simulink model "test_GRM_Airframe"  (R2019b)
settings: Solver=FixedStepAuto  StartTime=0.0  StopTime=60  FixedStep=0.001  RelTol=1e-3
PreLoadFcn:
  | addpath('init_functions');
  | init_grm;
  | addpath('parameters');
  | para_def_grm;
values from neighbouring files (symbols this model uses):
  a_vBEW = 0    [init_grm.m]
  act_dmp = 0.6322    [para_def_grm.m]
  act_omega = 59.9250    (= 59.925)    [para_def_grm.m]
  aero = load('aero.mat')    [para_def_grm.m]
  c_be = -6.5e-3    (= -0.0065)    [init_grm.m]
  c_h_geop0 = 0    [init_grm.m]
  c_h_geope = 11e3    (= 11000)    [init_grm.m]
  c_pa0 = 101325    [init_grm.m]
  c_pe = -c_g0/c_be/sgc    (= 5.25587981272)    [init_grm.m]
  c_r0 = 6371000.79    [init_grm.m]
  c_rot = 7.292115e-5    (= 7.292115e-05)    [init_grm.m]
  c_Tmp0 = 288.15    [init_grm.m]
  chW = pi/2    (= 1.57079632679)    [init_grm.m]
  D = JD - 2451545.0    [init_grm.m]
  d_siB_0 = 0    [para_def_grm.m]
  d_siB_max = deg2rad(1200)    [para_def_grm.m]
  d_siB_min = deg2rad(-1200)    [para_def_grm.m]
  dd_siB_max = deg2rad(50000)    [para_def_grm.m]
  dd_siB_min = deg2rad(-50000)    [para_def_grm.m]
  de_JBBB_xx = JBBB_xx_0 - JBBB_xx_e    (= 0)    [para_def_grm.m]
  de_JBBB_yy = JBBB_yy_0 - JBBB_yy_e    (= 0)    [para_def_grm.m]
  de_JBBB_zz = JBBB_zz_0 - JBBB_zz_e    (= 0)    [para_def_grm.m]
  de_mM = m_fuel_lookup(end)    [para_def_grm.m]
  e_pa = 0    [init_grm.m]
  e_Tmp = 0    [init_grm.m]
  F_prp = [450.52;428.7;423.25;391.61;352.34;304.35;266.17;243.26;216.92 ... (first row only)    [para_def_grm.m]
  flag_I_aero_switch = 1    [init_grm.m]
  flag_I_flat = 1    [init_grm.m]
  flag_I_gravity_switch = 1    [init_grm.m]
  flag_I_rot = 0    [init_grm.m]
  hcr = 1.4    [init_grm.m]
  J0PB_e = TBP*J0PP_e*TBP'    [para_def_grm.m]
  JMMM_0 = TBP*J0PP_0*TBP'    [para_def_grm.m]
  JMMM_e = TBP*J0PP_e*TBP'    [para_def_grm.m]
  lat_0 = 0    [init_grm.m]
  lon_0 = 0    [init_grm.m]
  m0 = mB_0    (= 3.30977)    [para_def_grm.m]
  m_fuel_lookup = [0;0.0573;0.1127;0.1667;0.2186;0.2681;0.3149;0.3588 ... (first row only)    [para_def_grm.m]
  mB_0 = 3.30977    [para_def_grm.m]
  mM_0 = 1.119    [para_def_grm.m]
  mM_e = de_mM    [para_def_grm.m]
  p0PB = [x0PB;y0PB;z0PB]    [para_def_grm.m]
  pBII_0 = TIE_0*pBEE_0    [init_grm.m]
  pMPB = [xMPB;yMPB;zMPB]    [para_def_grm.m]
  pNPB = [0;0;0]    [para_def_grm.m]
  qEG_0 = q12_from_T12(TEG)    [init_grm.m]
  qIB_0 = qumul(qIG_0,qGB_0)    [init_grm.m]
  qIE_0 = q12_from_T12(TIE_0)    [init_grm.m]
  sgc = 287.05287    [init_grm.m]
  siB_0 = 0    [para_def_grm.m]
  siB_max = deg2rad(30)    [para_def_grm.m]
  siB_min = deg2rad(-30)    [para_def_grm.m]
  t_prp1 = [0.04;0.28;0.54;1;1.48;1.99;2.51;3;3.5;3.67;3.82;4]    [para_def_grm.m]
  t_prp2 = t_prp2'    [para_def_grm.m]
  T_sim_lnch = -5    [init_grm.m]
  Tr3r4 = [1,1,1,1;1,1,-1,-1;-1,1,1,-1]*0.25    [para_def_grm.m]
  Tr4r3 = [1,1,-1;1,1,1;1,-1,1;1,-1,-1]    [para_def_grm.m]
  tRRR = 0    [para_def_grm.m]
  unc_a_vBEW_bl = 0    [para_def_grm.m]
  unc_act_bl = 0    [para_def_grm.m]
  unc_act_off = 0    [para_def_grm.m]
  unc_act_scale = 1    [para_def_grm.m]
  unc_aero_Cl_scale = 1    [para_def_grm.m]
  unc_aero_Cm_scale = 1    [para_def_grm.m]
  unc_aero_Cn_scale = 1    [para_def_grm.m]
  unc_aero_Cx_scale = 1    [para_def_grm.m]
  unc_aero_Cy_scale = 1    [para_def_grm.m]
  unc_aero_Cz_scale = 1    [para_def_grm.m]
  unc_cg_x = 0    [para_def_grm.m]
  unc_cg_y = 0    [para_def_grm.m]
  unc_cg_z = 0    [para_def_grm.m]
  unc_chW_bl = 0    [para_def_grm.m]
  unc_fin_def_pitch = 0    [para_def_grm.m]
  unc_fin_def_roll = 0    [para_def_grm.m]
  unc_fin_def_yaw = 0    [para_def_grm.m]
  unc_mB_bl = 0    [para_def_grm.m]
  unc_mB_scale = 1    [para_def_grm.m]
  unc_moi_Jxx = 0    [para_def_grm.m]
  unc_moi_Jyy = 0    [para_def_grm.m]
  unc_moi_Jzz = 0    [para_def_grm.m]
  unc_prp_scale = 1    [para_def_grm.m]
  unc_prp_x = 0    [para_def_grm.m]
  unc_prp_y = 0    [para_def_grm.m]
  unc_prp_z = 0    [para_def_grm.m]
  vBII_0 = vBEE_0 + cross(wIEI_0,pBII_0)    [init_grm.m]
  wBIB_0 = r2_from_r1_trans_q21(wBII_0,qBI_0)    [init_grm.m]
  x0PB = -0.5    [para_def_grm.m]
  xMPB = -0.9    [para_def_grm.m]
  y0PB = 0    [para_def_grm.m]
  yMPB = 0    [para_def_grm.m]
  z0PB = 0    [para_def_grm.m]
  zMPB = 0    [para_def_grm.m]
undefined symbols (not defined in the file or in its folder): c_b_WGS, c_flat, c_grav, c_rsma, d_mB_lookup, t_dmB
libraries: simulink_extras x14, simulink x3
(part 6 of 6)

== system test_GRM_Airframe/GRM_Airframe/rb_eom/eom_6dof/Rigid_Body_EOM_6_DOF/rb_eom_6dof/r2_from_r1_trans_q21 ==
  note: Outputs [size]:
      |
      | vector r2 [3]
  note: Inputs [size]:
      |
      | vector r1 [3]
      | quaternion q21 [4]
  r1 : Inport
  q21 : Inport  Port=2
  Add : Sum  Inputs=++++
  Add1 : Sum  Inputs=++++
  Constant : Constant  Value=0
  Demux : Demux  Outputs=3
  Demux1 : Demux
  Demux2 : Demux
  Math Function : Math  Operator=transpose  SaturateOnIntegerOverflow=on
  Product{,1..7} (8 alike) : Product
  Product8 : Product  Inputs=3  Multiplication=Matrix(*)
  Q_1 : Constant  Value=[0 0 0 1; 0 0 1 0; 0 -1 0 0; -1 0 0 0]
  Q_2 : Constant  Value=[0 0 -1 0; 0 0 0 1; 1 0 0 0; 0 -1 0 0]
  Q_3 : Constant  Value=[0 1 0 0; -1 0 0 0; 0 0 0 1; 0 0 -1 0]
  Q_4 : Constant  Value=[1 0 0 0; 0 1 0 0; 0 0 1 0; 0 0 0 1]
  Q~_1 : Constant  Value=[0 0 0 1; 0 0 -1 0; 0 1 0 0; -1 0 0 0]
  Q~_2 : Constant  Value=[0 0 1 0; 0 0 0 1; -1 0 0 0; 0 -1 0 0]
  Q~_3 : Constant  Value=[0 -1 0 0; 1 0 0 0; 0 0 0 1; 0 0 -1 0]
  Q~_4 : Constant  Value=[1 0 0 0; 0 1 0 0; 0 0 1 0; 0 0 0 1]
  Selector : Selector  IndexMode=Zero-based  InputPortWidth=4  IndexOptions=Index vector (dialog)  Indices=[0 1 2]  OutputSizes=1
  Vector Concatenate : Concatenate  NumInputs=4
  r2 : Outport  VectorParamsAs1DForOutWhenUnconnected=off
  wires:
  Selector/1 -> r2/1
  Product8/1 -> Selector/1
  Vector Concatenate/1 -> Product8/3
  Constant/1 -> Vector Concatenate/4
  Math Function/1 -> Product8/1  "Q~T(q)"
  Q~_3/1 -> Product6/1
  Q~_1/1 -> Product4/1
  Q~_4/1 -> Product7/1
  Product6/1 -> Add1/3
  Demux2/3 -> Product6/2  "q3"
  Product5/1 -> Add1/2
  Demux2/2 -> Product5/2  "q2"
  Add1/1 -> Math Function/1  "Q~(q)"
  q21/1 -> Demux1/1, Demux2/1
  Product7/1 -> Add1/4
  Product4/1 -> Add1/1
  Q~_2/1 -> Product5/1
  Demux2/4 -> Product7/2  "q4"
  Demux2/1 -> Product4/2  "q1"
  Add/1 -> Product8/2  "Q(q)"
  Product3/1 -> Add/4
  Product2/1 -> Add/3
  Product1/1 -> Add/2
  Product/1 -> Add/1
  Q_4/1 -> Product3/1
  Q_3/1 -> Product2/1
  Q_2/1 -> Product1/1
  Q_1/1 -> Product/1
  Demux1/4 -> Product3/2  "q4"
  Demux1/3 -> Product2/2  "q3"
  Demux1/2 -> Product1/2  "q2"
  Demux1/1 -> Product/2  "q1"
  Demux/3 -> Vector Concatenate/3  "rz"
  Demux/2 -> Vector Concatenate/2  "ry"
  Demux/1 -> Vector Concatenate/1  "rx"
  r1/1 -> Demux/1

== system test_GRM_Airframe/GRM_Airframe/stream_flow/calc_stream_flow/Subsystem1/AoA_Sideslip_Alphatot_Phi/norm_of_vector ==
  note: Outputs [size]:
      |
      | norm of vector [1]
  note: Inputs [size]:
      |
      | vector  [3]
  vector : Inport
  Dot Product1 : DotProduct  InputSameDT=on  OutDataTypeStr=Inherit: Inherit via internal rule
  Math Function1 : Math  Operator=sqrt  SaturateOnIntegerOverflow=on
  norm_of_vector : Outport  VectorParamsAs1DForOutWhenUnconnected=off
  wires:
  vector/1 -> Dot Product1/1, Dot Product1/2
  Math Function1/1 -> norm_of_vector/1
  Dot Product1/1 -> Math Function1/1

== system test_GRM_Airframe/GRM_Airframe/weight_and_balance/moi/moi_coordinate_transformation/3_rot_mat/1. Rotation x-Achse ==
  alpha1 : Inport
  Constant : Constant
  Constant{1..2,7..8} (4 alike) : Constant  Value=0
  Gain : Gain  Gain=-1
  Matrix Concatenate : Concatenate  NumInputs=3  Mode=Multidimensional array  ConcatenateDimension=2
  Mux : Mux  Inputs=3
  Mux1 : Mux  Inputs=3
  Mux2 : Mux  Inputs=3
  Trigonometric Function : Trigonometry  Operator=cos
  Trigonometric Function1 : Trigonometry
  Trigonometric Function2 : Trigonometry
  Trigonometric Function3 : Trigonometry  Operator=cos
  1Rot_Matrix_x : Outport  VectorParamsAs1DForOutWhenUnconnected=off
  wires:
  Gain/1 -> Mux1/3
  alpha1/1 -> Trigonometric Function2/1, Trigonometric Function/1, Trigonometric Function1/1, Trigonometric Function3/1
  Constant/1 -> Mux/1
  Constant1/1 -> Mux/2
  Constant2/1 -> Mux/3
  Constant8/1 -> Mux1/1
  Trigonometric Function/1 -> Mux1/2
  Trigonometric Function2/1 -> Gain/1
  Constant7/1 -> Mux2/1
  Trigonometric Function1/1 -> Mux2/2
  Trigonometric Function3/1 -> Mux2/3
  Mux/1 -> Matrix Concatenate/1
  Mux1/1 -> Matrix Concatenate/2
  Mux2/1 -> Matrix Concatenate/3
  Matrix Concatenate/1 -> 1Rot_Matrix_x/1

== system test_GRM_Airframe/GRM_Airframe/weight_and_balance/moi/moi_coordinate_transformation/3_rot_mat/1. Rotation y-Achse ==
  alpha1 : Inport
  Constant{,2,7..8} (4 alike) : Constant  Value=0
  Constant1 : Constant
  Gain1 : Gain  Gain=-1
  Matrix Concatenate : Concatenate  NumInputs=3  Mode=Multidimensional array  ConcatenateDimension=2
  Mux : Mux  Inputs=3
  Mux1 : Mux  Inputs=3
  Mux2 : Mux  Inputs=3
  Trigonometric Function : Trigonometry  Operator=cos
  Trigonometric Function1 : Trigonometry
  Trigonometric Function2 : Trigonometry
  Trigonometric Function3 : Trigonometry  Operator=cos
  1Rot_Matrix_y : Outport  VectorParamsAs1DForOutWhenUnconnected=off
  wires:
  Gain1/1 -> Mux2/1
  Mux2/1 -> Matrix Concatenate/3
  Mux1/1 -> Matrix Concatenate/2
  Mux/1 -> Matrix Concatenate/1
  Trigonometric Function3/1 -> Mux2/3
  Trigonometric Function1/1 -> Gain1/1
  Constant2/1 -> Mux1/3
  Constant1/1 -> Mux1/2
  Constant/1 -> Mux1/1
  alpha1/1 -> Trigonometric Function1/1, Trigonometric Function3/1, Trigonometric Function2/1, Trigonometric Function/1
  Constant8/1 -> Mux/2
  Trigonometric Function/1 -> Mux/1
  Trigonometric Function2/1 -> Mux/3
  Constant7/1 -> Mux2/2
  Matrix Concatenate/1 -> 1Rot_Matrix_y/1

== system test_GRM_Airframe/GRM_Airframe/weight_and_balance/moi/moi_coordinate_transformation/3_rot_mat/1. Rotation z-Achse ==
  alpha1 : Inport
  Constant{4,7..8,10} (4 alike) : Constant  Value=0
  Constant11 : Constant
  Gain : Gain  Gain=-1
  Matrix Concatenate : Concatenate  NumInputs=3  Mode=Multidimensional array  ConcatenateDimension=2
  Mux : Mux  Inputs=3
  Mux1 : Mux  Inputs=3
  Mux2 : Mux  Inputs=3
  Trigonometric Function : Trigonometry  Operator=cos
  Trigonometric Function1 : Trigonometry
  Trigonometric Function3 : Trigonometry  Operator=cos
  Trigonometric Function4 : Trigonometry
  1Rot_Matrix_z : Outport  VectorParamsAs1DForOutWhenUnconnected=off
  wires:
  Gain/1 -> Mux/2
  Trigonometric Function/1 -> Mux1/2
  Mux/1 -> Matrix Concatenate/1
  Mux1/1 -> Matrix Concatenate/2
  Mux2/1 -> Matrix Concatenate/3
  Trigonometric Function1/1 -> Mux1/1
  Constant7/1 -> Mux1/3
  Constant4/1 -> Mux2/1
  Constant10/1 -> Mux2/2
  Constant11/1 -> Mux2/3
  Trigonometric Function3/1 -> Mux/1
  Trigonometric Function4/1 -> Gain/1
  Constant8/1 -> Mux/3
  Matrix Concatenate/1 -> 1Rot_Matrix_z/1
  alpha1/1 -> Trigonometric Function3/1, Trigonometric Function4/1, Trigonometric Function/1, Trigonometric Function1/1

== system test_GRM_Airframe/GRM_Airframe/weight_and_balance/moi/moi_coordinate_transformation/3_rot_mat/2. Rotation x-Achse ==
  alpha2 : Inport
  Constant : Constant
  Constant{1..2,7..8} (4 alike) : Constant  Value=0
  Gain : Gain  Gain=-1
  Matrix Concatenate : Concatenate  NumInputs=3  Mode=Multidimensional array  ConcatenateDimension=2
  Mux : Mux  Inputs=3
  Mux1 : Mux  Inputs=3
  Mux2 : Mux  Inputs=3
  Trigonometric Function : Trigonometry  Operator=cos
  Trigonometric Function1 : Trigonometry
  Trigonometric Function2 : Trigonometry
  Trigonometric Function3 : Trigonometry  Operator=cos
  2Rot_Matrix_x : Outport  VectorParamsAs1DForOutWhenUnconnected=off
  wires:
  Gain/1 -> Mux1/3
  alpha2/1 -> Trigonometric Function2/1, Trigonometric Function/1, Trigonometric Function1/1, Trigonometric Function3/1
  Constant/1 -> Mux/1
  Constant1/1 -> Mux/2
  Constant2/1 -> Mux/3
  Constant8/1 -> Mux1/1
  Trigonometric Function/1 -> Mux1/2
  Trigonometric Function2/1 -> Gain/1
  Constant7/1 -> Mux2/1
  Trigonometric Function1/1 -> Mux2/2
  Trigonometric Function3/1 -> Mux2/3
  Mux/1 -> Matrix Concatenate/1
  Mux1/1 -> Matrix Concatenate/2
  Mux2/1 -> Matrix Concatenate/3
  Matrix Concatenate/1 -> 2Rot_Matrix_x/1

== system test_GRM_Airframe/GRM_Airframe/weight_and_balance/moi/moi_coordinate_transformation/3_rot_mat/2. Rotation y-Achse ==
  alpha2 : Inport
  Constant{,2,7..8} (4 alike) : Constant  Value=0
  Constant1 : Constant
  Gain1 : Gain  Gain=-1
  Matrix Concatenate : Concatenate  NumInputs=3  Mode=Multidimensional array  ConcatenateDimension=2
  Mux : Mux  Inputs=3
  Mux1 : Mux  Inputs=3
  Mux2 : Mux  Inputs=3
  Trigonometric Function : Trigonometry  Operator=cos
  Trigonometric Function1 : Trigonometry
  Trigonometric Function2 : Trigonometry
  Trigonometric Function3 : Trigonometry  Operator=cos
  2Rot_Matrix_y : Outport  VectorParamsAs1DForOutWhenUnconnected=off
  wires:
  Gain1/1 -> Mux2/1
  Mux2/1 -> Matrix Concatenate/3
  Mux1/1 -> Matrix Concatenate/2
  Mux/1 -> Matrix Concatenate/1
  Trigonometric Function3/1 -> Mux2/3
  Trigonometric Function1/1 -> Gain1/1
  Constant2/1 -> Mux1/3
  Constant1/1 -> Mux1/2
  Constant/1 -> Mux1/1
  alpha2/1 -> Trigonometric Function1/1, Trigonometric Function3/1, Trigonometric Function2/1, Trigonometric Function/1
  Constant8/1 -> Mux/2
  Trigonometric Function/1 -> Mux/1
  Trigonometric Function2/1 -> Mux/3
  Constant7/1 -> Mux2/2
  Matrix Concatenate/1 -> 2Rot_Matrix_y/1

== system test_GRM_Airframe/GRM_Airframe/weight_and_balance/moi/moi_coordinate_transformation/3_rot_mat/2. Rotation z-Achse ==
  alpha2 : Inport
  Constant{4,7..8,10} (4 alike) : Constant  Value=0
  Constant11 : Constant
  Gain : Gain  Gain=-1
  Matrix Concatenate : Concatenate  NumInputs=3  Mode=Multidimensional array  ConcatenateDimension=2
  Mux : Mux  Inputs=3
  Mux1 : Mux  Inputs=3
  Mux2 : Mux  Inputs=3
  Trigonometric Function : Trigonometry  Operator=cos
  Trigonometric Function1 : Trigonometry
  Trigonometric Function3 : Trigonometry  Operator=cos
  Trigonometric Function4 : Trigonometry
  2Rot_Matrix_z : Outport  VectorParamsAs1DForOutWhenUnconnected=off
  wires:
  Gain/1 -> Mux/2
  Trigonometric Function/1 -> Mux1/2
  Mux/1 -> Matrix Concatenate/1
  Mux1/1 -> Matrix Concatenate/2
  Mux2/1 -> Matrix Concatenate/3
  Trigonometric Function1/1 -> Mux1/1
  Constant7/1 -> Mux1/3
  Constant4/1 -> Mux2/1
  Constant10/1 -> Mux2/2
  Constant11/1 -> Mux2/3
  Trigonometric Function3/1 -> Mux/1
  Trigonometric Function4/1 -> Gain/1
  Constant8/1 -> Mux/3
  Matrix Concatenate/1 -> 2Rot_Matrix_z/1
  alpha2/1 -> Trigonometric Function3/1, Trigonometric Function4/1, Trigonometric Function/1, Trigonometric Function1/1

== system test_GRM_Airframe/GRM_Airframe/weight_and_balance/moi/moi_coordinate_transformation/3_rot_mat/3. Rotation x-Achse ==
  alpha3 : Inport
  Constant : Constant
  Constant{1..2,7..8} (4 alike) : Constant  Value=0
  Gain : Gain  Gain=-1
  Matrix Concatenate : Concatenate  NumInputs=3  Mode=Multidimensional array  ConcatenateDimension=2
  Mux : Mux  Inputs=3
  Mux1 : Mux  Inputs=3
  Mux2 : Mux  Inputs=3
  Trigonometric Function : Trigonometry  Operator=cos
  Trigonometric Function1 : Trigonometry
  Trigonometric Function2 : Trigonometry
  Trigonometric Function3 : Trigonometry  Operator=cos
  3Rot_Matrix_x : Outport  VectorParamsAs1DForOutWhenUnconnected=off
  wires:
  Gain/1 -> Mux1/3
  alpha3/1 -> Trigonometric Function2/1, Trigonometric Function/1, Trigonometric Function1/1, Trigonometric Function3/1
  Constant/1 -> Mux/1
  Constant1/1 -> Mux/2
  Constant2/1 -> Mux/3
  Constant8/1 -> Mux1/1
  Trigonometric Function/1 -> Mux1/2
  Trigonometric Function2/1 -> Gain/1
  Constant7/1 -> Mux2/1
  Trigonometric Function1/1 -> Mux2/2
  Trigonometric Function3/1 -> Mux2/3
  Mux/1 -> Matrix Concatenate/1
  Mux1/1 -> Matrix Concatenate/2
  Mux2/1 -> Matrix Concatenate/3
  Matrix Concatenate/1 -> 3Rot_Matrix_x/1

== system test_GRM_Airframe/GRM_Airframe/weight_and_balance/moi/moi_coordinate_transformation/3_rot_mat/3. Rotation y-Achse ==
  alpha3 : Inport
  Constant{,2,7..8} (4 alike) : Constant  Value=0
  Constant1 : Constant
  Gain1 : Gain  Gain=-1
  Matrix Concatenate : Concatenate  NumInputs=3  Mode=Multidimensional array  ConcatenateDimension=2
  Mux : Mux  Inputs=3
  Mux1 : Mux  Inputs=3
  Mux2 : Mux  Inputs=3
  Trigonometric Function : Trigonometry  Operator=cos
  Trigonometric Function1 : Trigonometry
  Trigonometric Function2 : Trigonometry
  Trigonometric Function3 : Trigonometry  Operator=cos
  3Rot_Matrix_y : Outport  VectorParamsAs1DForOutWhenUnconnected=off
  wires:
  Gain1/1 -> Mux2/1
  Mux2/1 -> Matrix Concatenate/3
  Mux1/1 -> Matrix Concatenate/2
  Mux/1 -> Matrix Concatenate/1
  Trigonometric Function3/1 -> Mux2/3
  Trigonometric Function1/1 -> Gain1/1
  Constant2/1 -> Mux1/3
  Constant1/1 -> Mux1/2
  Constant/1 -> Mux1/1
  alpha3/1 -> Trigonometric Function1/1, Trigonometric Function3/1, Trigonometric Function2/1, Trigonometric Function/1
  Constant8/1 -> Mux/2
  Trigonometric Function/1 -> Mux/1
  Trigonometric Function2/1 -> Mux/3
  Constant7/1 -> Mux2/2
  Matrix Concatenate/1 -> 3Rot_Matrix_y/1

== system test_GRM_Airframe/GRM_Airframe/weight_and_balance/moi/moi_coordinate_transformation/3_rot_mat/3. Rotation z-Achse ==
  alpha3 : Inport
  Constant{4,7..8,10} (4 alike) : Constant  Value=0
  Constant11 : Constant
  Gain : Gain  Gain=-1
  Matrix Concatenate : Concatenate  NumInputs=3  Mode=Multidimensional array  ConcatenateDimension=2
  Mux : Mux  Inputs=3
  Mux1 : Mux  Inputs=3
  Mux2 : Mux  Inputs=3
  Trigonometric Function : Trigonometry  Operator=cos
  Trigonometric Function1 : Trigonometry
  Trigonometric Function3 : Trigonometry  Operator=cos
  Trigonometric Function4 : Trigonometry
  3Rot_Matrix_z : Outport  VectorParamsAs1DForOutWhenUnconnected=off
  wires:
  Gain/1 -> Mux/2
  Trigonometric Function/1 -> Mux1/2
  Mux/1 -> Matrix Concatenate/1
  Mux1/1 -> Matrix Concatenate/2
  Mux2/1 -> Matrix Concatenate/3
  Trigonometric Function1/1 -> Mux1/1
  Constant7/1 -> Mux1/3
  Constant4/1 -> Mux2/1
  Constant10/1 -> Mux2/2
  Constant11/1 -> Mux2/3
  Trigonometric Function3/1 -> Mux/1
  Trigonometric Function4/1 -> Gain/1
  Constant8/1 -> Mux/3
  Matrix Concatenate/1 -> 3Rot_Matrix_z/1
  alpha3/1 -> Trigonometric Function3/1, Trigonometric Function4/1, Trigonometric Function/1, Trigonometric Function1/1

== system test_GRM_Airframe/environment_global/weather/atm_dynamic/trafo_around_z_axis/1_rot_mat/1. Rotation x-Achse ==
  alpha1 : Inport
  Constant : Constant
  Constant{1..2,7..8} (4 alike) : Constant  Value=0
  Gain : Gain  Gain=-1
  Matrix Concatenate : Concatenate  NumInputs=3  Mode=Multidimensional array  ConcatenateDimension=2
  Mux : Mux  Inputs=3
  Mux1 : Mux  Inputs=3
  Mux2 : Mux  Inputs=3
  Trigonometric Function : Trigonometry  Operator=cos
  Trigonometric Function1 : Trigonometry
  Trigonometric Function2 : Trigonometry
  Trigonometric Function3 : Trigonometry  Operator=cos
  1Rot_Matrix_x : Outport  VectorParamsAs1DForOutWhenUnconnected=off
  wires:
  Gain/1 -> Mux1/3
  Matrix Concatenate/1 -> 1Rot_Matrix_x/1
  Mux2/1 -> Matrix Concatenate/3
  Mux1/1 -> Matrix Concatenate/2
  Mux/1 -> Matrix Concatenate/1
  Trigonometric Function3/1 -> Mux2/3
  Trigonometric Function1/1 -> Mux2/2
  Constant7/1 -> Mux2/1
  Trigonometric Function2/1 -> Gain/1
  Trigonometric Function/1 -> Mux1/2
  Constant8/1 -> Mux1/1
  Constant2/1 -> Mux/3
  Constant1/1 -> Mux/2
  Constant/1 -> Mux/1
  alpha1/1 -> Trigonometric Function3/1, Trigonometric Function1/1, Trigonometric Function/1, Trigonometric Function2/1

== system test_GRM_Airframe/environment_global/weather/atm_dynamic/trafo_around_z_axis/1_rot_mat/1. Rotation y-Achse ==
  alpha1 : Inport
  Constant{,2,7..8} (4 alike) : Constant  Value=0
  Constant1 : Constant
  Gain1 : Gain  Gain=-1
  Matrix Concatenate : Concatenate  NumInputs=3  Mode=Multidimensional array  ConcatenateDimension=2
  Mux : Mux  Inputs=3
  Mux1 : Mux  Inputs=3
  Mux2 : Mux  Inputs=3
  Trigonometric Function : Trigonometry  Operator=cos
  Trigonometric Function1 : Trigonometry
  Trigonometric Function2 : Trigonometry
  Trigonometric Function3 : Trigonometry  Operator=cos
  1Rot_Matrix_y : Outport  VectorParamsAs1DForOutWhenUnconnected=off
  wires:
  Gain1/1 -> Mux2/1
  Matrix Concatenate/1 -> 1Rot_Matrix_y/1
  Constant7/1 -> Mux2/2
  Trigonometric Function2/1 -> Mux/3
  Trigonometric Function/1 -> Mux/1
  Constant8/1 -> Mux/2
  alpha1/1 -> Trigonometric Function/1, Trigonometric Function2/1, Trigonometric Function3/1, Trigonometric Function1/1
  Constant/1 -> Mux1/1
  Constant1/1 -> Mux1/2
  Constant2/1 -> Mux1/3
  Trigonometric Function1/1 -> Gain1/1
  Trigonometric Function3/1 -> Mux2/3
  Mux/1 -> Matrix Concatenate/1
  Mux1/1 -> Matrix Concatenate/2
  Mux2/1 -> Matrix Concatenate/3

== system test_GRM_Airframe/environment_global/weather/atm_dynamic/trafo_around_z_axis/1_rot_mat/1. Rotation z-Achse ==
  alpha1 : Inport
  Constant{4,7..8,10} (4 alike) : Constant  Value=0
  Constant11 : Constant
  Gain : Gain  Gain=-1
  Matrix Concatenate : Concatenate  NumInputs=3  Mode=Multidimensional array  ConcatenateDimension=2
  Mux : Mux  Inputs=3
  Mux1 : Mux  Inputs=3
  Mux2 : Mux  Inputs=3
  Trigonometric Function : Trigonometry  Operator=cos
  Trigonometric Function1 : Trigonometry
  Trigonometric Function3 : Trigonometry  Operator=cos
  Trigonometric Function4 : Trigonometry
  1Rot_Matrix_z : Outport  VectorParamsAs1DForOutWhenUnconnected=off
  wires:
  Gain/1 -> Mux/2
  alpha1/1 -> Trigonometric Function1/1, Trigonometric Function/1, Trigonometric Function4/1, Trigonometric Function3/1
  Matrix Concatenate/1 -> 1Rot_Matrix_z/1
  Constant8/1 -> Mux/3
  Trigonometric Function4/1 -> Gain/1
  Trigonometric Function3/1 -> Mux/1
  Constant11/1 -> Mux2/3
  Constant10/1 -> Mux2/2
  Constant4/1 -> Mux2/1
  Constant7/1 -> Mux1/3
  Trigonometric Function1/1 -> Mux1/1
  Mux2/1 -> Matrix Concatenate/3
  Mux1/1 -> Matrix Concatenate/2
  Mux/1 -> Matrix Concatenate/1
  Trigonometric Function/1 -> Mux1/2

== system test_GRM_Airframe/GRM_Airframe/aerodynamics/aerodynamic_via_lookup/calc_aero_for_mom/launch_rail/initial_altitude/trafo_E_to_geodetic ==
  note: Outputs [size]:
      |
      | geodetic longitude [1]
      | geodetic latitude [1]
      | geodetic altitude [1]
  note: Inputs [size]:
      |
      | position_E [3]
  pBEE : Inport
  Geodetic_altitude : Subsystem
  Geodetic_latitude : Subsystem
  Selector1 : Selector  IndexMode=Zero-based  InputPortWidth=3  IndexOptions=Index vector (dialog)  Indices=1  OutputSizes=1
  Selector2 : Selector  IndexMode=Zero-based  InputPortWidth=3  IndexOptions=Index vector (dialog)  Indices=0  OutputSizes=1
  Trigonometric Function1 : Trigonometry  Operator=atan2
  c_flat : Constant  Value=c_flat
  c_rsma : Constant  Value=c_rsma
  lon : Outport  VectorParamsAs1DForOutWhenUnconnected=off
  lat : Outport  Port=2  VectorParamsAs1DForOutWhenUnconnected=off
  alt : Outport  Port=3  VectorParamsAs1DForOutWhenUnconnected=off
  wires:
  c_flat/1 -> Geodetic_altitude/3(c_flat), Geodetic_latitude/3(c_flat)  "c_flat"
  c_rsma/1 -> Geodetic_latitude/2(c_rsma), Geodetic_altitude/2(c_rsma)  "c_rsma"
  Selector1/1 -> Trigonometric Function1/1  "pBEE_y"
  Selector2/1 -> Trigonometric Function1/2  "pBEE_x"
  Geodetic_latitude/1(lat) -> Geodetic_altitude/4(lat), lat/1
  Geodetic_altitude/1(alt) -> alt/1
  Trigonometric Function1/1 -> lon/1  "lon"
  pBEE/1 -> Selector1/1, Selector2/1, Geodetic_latitude/1(pBEE), Geodetic_altitude/1(pBEE)  "pBEE"

== system test_GRM_Airframe/GRM_Airframe/aerodynamics/aerodynamic_via_lookup/calc_aero_for_mom/launch_rail1/initial_altitude/trafo_E_to_geodetic ==
  note: Outputs [size]:
      |
      | geodetic longitude [1]
      | geodetic latitude [1]
      | geodetic altitude [1]
  note: Inputs [size]:
      |
      | position_E [3]
  pBEE : Inport
  Geodetic_altitude : Subsystem
  Geodetic_latitude : Subsystem
  Selector1 : Selector  IndexMode=Zero-based  InputPortWidth=3  IndexOptions=Index vector (dialog)  Indices=1  OutputSizes=1
  Selector2 : Selector  IndexMode=Zero-based  InputPortWidth=3  IndexOptions=Index vector (dialog)  Indices=0  OutputSizes=1
  Trigonometric Function1 : Trigonometry  Operator=atan2
  c_flat : Constant  Value=c_flat
  c_rsma : Constant  Value=c_rsma
  lon : Outport  VectorParamsAs1DForOutWhenUnconnected=off
  lat : Outport  Port=2  VectorParamsAs1DForOutWhenUnconnected=off
  alt : Outport  Port=3  VectorParamsAs1DForOutWhenUnconnected=off
  wires:
  c_flat/1 -> Geodetic_altitude/3(c_flat), Geodetic_latitude/3(c_flat)  "c_flat"
  c_rsma/1 -> Geodetic_latitude/2(c_rsma), Geodetic_altitude/2(c_rsma)  "c_rsma"
  Selector1/1 -> Trigonometric Function1/1  "pBEE_y"
  Selector2/1 -> Trigonometric Function1/2  "pBEE_x"
  Geodetic_latitude/1(lat) -> Geodetic_altitude/4(lat), lat/1
  Geodetic_altitude/1(alt) -> alt/1
  Trigonometric Function1/1 -> lon/1  "lon"
  pBEE/1 -> Selector1/1, Selector2/1, Geodetic_latitude/1(pBEE), Geodetic_altitude/1(pBEE)  "pBEE"

== system test_GRM_Airframe/GRM_Airframe/motion_kinematics/calc_motion_kinematics/earth_rotation/quaternion_integration/Subsystem1/conjugate_quaternion1 ==
  note: Outputs [size]:
      |
      | q_conj [4]
  note: Inputs [size]:
      |
      | q [4]
  q : Inport
  Demux : Demux  Outputs=[3;1]
  Gain1 : Gain  Gain=-1
  Vector Concatenate : Concatenate
  q_conj : Outport  VectorParamsAs1DForOutWhenUnconnected=off
  wires:
  Demux/2 -> Vector Concatenate/2
  Gain1/1 -> Vector Concatenate/1
  Demux/1 -> Gain1/1
  Vector Concatenate/1 -> q_conj/1
  q/1 -> Demux/1

== system test_GRM_Airframe/GRM_Airframe/motion_kinematics/calc_motion_kinematics/earth_rotation/quaternion_integration/Subsystem1/conjugate_quaternion2 ==
  note: Outputs [size]:
      |
      | q_conj [4]
  note: Inputs [size]:
      |
      | q [4]
  q : Inport
  Demux : Demux  Outputs=[3;1]
  Gain1 : Gain  Gain=-1
  Vector Concatenate : Concatenate
  q_conj : Outport  VectorParamsAs1DForOutWhenUnconnected=off
  wires:
  Demux/2 -> Vector Concatenate/2
  Gain1/1 -> Vector Concatenate/1
  Demux/1 -> Gain1/1
  Vector Concatenate/1 -> q_conj/1
  q/1 -> Demux/1

== system test_GRM_Airframe/GRM_Airframe/motion_kinematics/calc_motion_kinematics/earth_rotation/quaternion_integration1/Subsystem1/conjugate_quaternion1 ==
  note: Outputs [size]:
      |
      | q_conj [4]
  note: Inputs [size]:
      |
      | q [4]
  q : Inport
  Demux : Demux  Outputs=[3;1]
  Gain1 : Gain  Gain=-1
  Vector Concatenate : Concatenate
  q_conj : Outport  VectorParamsAs1DForOutWhenUnconnected=off
  wires:
  Demux/2 -> Vector Concatenate/2
  Gain1/1 -> Vector Concatenate/1
  Demux/1 -> Gain1/1
  Vector Concatenate/1 -> q_conj/1
  q/1 -> Demux/1

== system test_GRM_Airframe/GRM_Airframe/motion_kinematics/calc_motion_kinematics/earth_rotation/quaternion_integration1/Subsystem1/conjugate_quaternion2 ==
  note: Outputs [size]:
      |
      | q_conj [4]
  note: Inputs [size]:
      |
      | q [4]
  q : Inport
  Demux : Demux  Outputs=[3;1]
  Gain1 : Gain  Gain=-1
  Vector Concatenate : Concatenate
  q_conj : Outport  VectorParamsAs1DForOutWhenUnconnected=off
  wires:
  Demux/2 -> Vector Concatenate/2
  Gain1/1 -> Vector Concatenate/1
  Demux/1 -> Gain1/1
  Vector Concatenate/1 -> q_conj/1
  q/1 -> Demux/1

== system test_GRM_Airframe/GRM_Airframe/rb_eom/eom_6dof/Rigid_Body_EOM_6_DOF/rb_eom_6dof/calc_d_qIB/conjugate_quaternion ==
  note: Outputs [size]:
      |
      | q_conj [4]
  note: Inputs [size]:
      |
      | q [4]
  q : Inport
  Demux : Demux  Outputs=[3;1]
  Gain1 : Gain  Gain=-1
  Vector Concatenate : Concatenate
  q_conj : Outport  VectorParamsAs1DForOutWhenUnconnected=off
  wires:
  Demux/2 -> Vector Concatenate/2
  Gain1/1 -> Vector Concatenate/1
  Demux/1 -> Gain1/1
  Vector Concatenate/1 -> q_conj/1
  q/1 -> Demux/1

== system test_GRM_Airframe/GRM_Airframe/rb_eom/eom_6dof/Rigid_Body_EOM_6_DOF/rb_eom_6dof/calc_d_qIB/conjugate_quaternion1 ==
  note: Outputs [size]:
      |
      | q_conj [4]
  note: Inputs [size]:
      |
      | q [4]
  q : Inport
  Demux : Demux  Outputs=[3;1]
  Gain1 : Gain  Gain=-1
  Vector Concatenate : Concatenate
  q_conj : Outport  VectorParamsAs1DForOutWhenUnconnected=off
  wires:
  Demux/2 -> Vector Concatenate/2
  Gain1/1 -> Vector Concatenate/1
  Demux/1 -> Gain1/1
  Vector Concatenate/1 -> q_conj/1
  q/1 -> Demux/1

== system test_GRM_Airframe/GRM_Airframe/aerodynamics/aerodynamic_via_lookup/calc_aero_for_mom/launch_rail/initial_altitude/trafo_E_to_geodetic/Geodetic_altitude ==
  pBEE : Inport
  c_rsma : Inport  Port=2
  c_flat : Inport  Port=3
  lat : Inport  Port=4
  Add : Sum
  Constant : Constant
  Gain : Gain  Gain=2
  Product : Product  Inputs=*/  SaturateOnIntegerOverflow=on  RndMeth=Zero  InputSameDT=on  OutDataTypeStr=Inherit: Same as first input
  Product1 : Product
  Product2 : Product
  Product3 : Product
  Product4 : Product  Inputs=*/  SaturateOnIntegerOverflow=on  RndMeth=Zero  InputSameDT=on  OutDataTypeStr=Inherit: Same as first input
  Product5 : Product  Inputs=3
  Selector : Selector  IndexMode=Zero-based  InputPortWidth=3  IndexOptions=Index vector (dialog)  Indices=0  OutputSizes=1
  Selector1 : Selector  IndexMode=Zero-based  InputPortWidth=3  IndexOptions=Index vector (dialog)  Indices=1  OutputSizes=1
  Sqrt : Sqrt  SaturateOnIntegerOverflow=on
  Sqrt1 : Sqrt  SaturateOnIntegerOverflow=on
  Subtract : Sum  Inputs=+-
  Subtract1 : Sum  Inputs=+-
  Sum : Sum  Inputs=+-  SaturateOnIntegerOverflow=on  InputSameDT=on  OutDataTypeStr=Inherit: Same as first input
  Trigonometric Function : Trigonometry
  cos(latGD) : Trigonometry  Operator=cos
  alt : Outport  VectorParamsAs1DForOutWhenUnconnected=off
  wires:
  Product4/1 -> Sum/2
  Trigonometric Function/1 -> Product5/1, Product5/2
  Product5/1 -> Subtract1/2
  Constant/1 -> Subtract1/1
  Subtract1/1 -> Sqrt1/1
  Sqrt1/1 -> Product4/2
  c_flat/1 -> Gain/1, Product3/2, Product3/1
  Gain/1 -> Subtract/1
  Product3/1 -> Subtract/2
  pBEE/1 -> Selector/1, Selector1/1
  Add/1 -> Sqrt/1
  Product2/1 -> Add/2
  Product1/1 -> Add/1
  Selector1/1 -> Product2/1, Product2/2
  Selector/1 -> Product1/1, Product1/2
  Sum/1 -> alt/1  "alt"
  Product/1 -> Sum/1
  Subtract/1 -> Product5/3
  c_rsma/1 -> Product4/1
  cos(latGD)/1 -> Product/2
  Sqrt/1 -> Product/1
  lat/1 -> cos(latGD)/1, Trigonometric Function/1

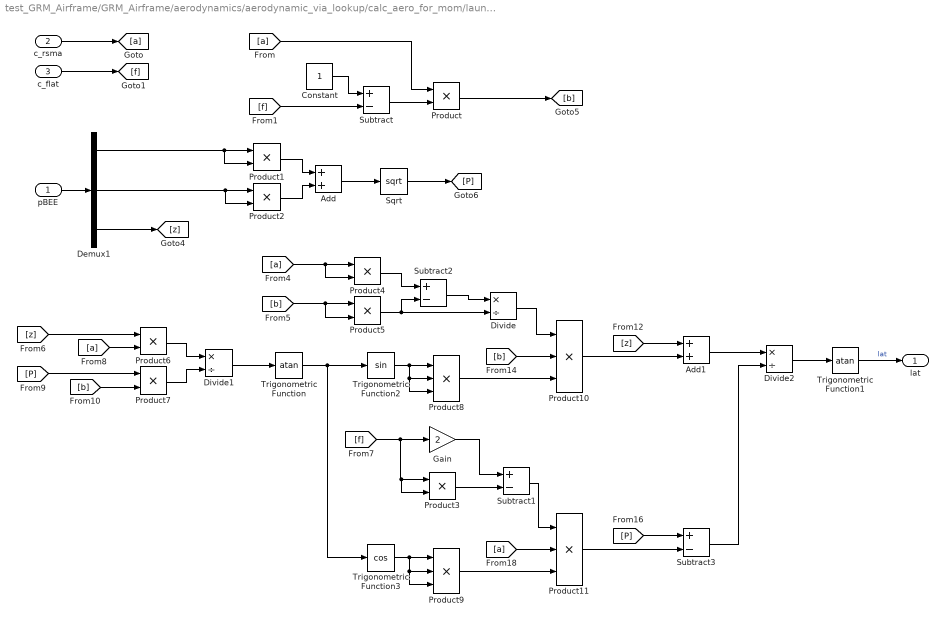
== system test_GRM_Airframe/GRM_Airframe/aerodynamics/aerodynamic_via_lookup/calc_aero_for_mom/launch_rail/initial_altitude/trafo_E_to_geodetic/Geodetic_latitude ==
  pBEE : Inport
  c_rsma : Inport  Port=2
  c_flat : Inport  Port=3
  Add : Sum
  Add1 : Sum
  Constant : Constant
  Demux1 : Demux  Outputs=[1;1;1]
  Divide : Product  Inputs=*/
  Divide1 : Product  Inputs=*/
  Divide2 : Product  Inputs=*/
  Gain : Gain  Gain=2
  Product{,1..7} (8 alike) : Product
  Product{8..11} (4 alike) : Product  Inputs=3
  Sqrt : Sqrt  SaturateOnIntegerOverflow=on
  Subtract{,1..3} (4 alike) : Sum  Inputs=+-
  Trigonometric Function : Trigonometry  Operator=atan
  Trigonometric Function1 : Trigonometry  Operator=atan
  Trigonometric Function2 : Trigonometry
  Trigonometric Function3 : Trigonometry  Operator=cos
  lat : Outport  VectorParamsAs1DForOutWhenUnconnected=off
  wires:
  Divide/1 -> Product10/1
  Product9/1 -> Product11/3
  Product11/1 -> Subtract3/2
  Subtract3/1 -> Divide2/2
  Add1/1 -> Divide2/1
  Product10/1 -> Add1/2
  Product8/1 -> Product10/3
  Trigonometric Function3/1 -> Product9/1, Product9/3, Product9/2
  Trigonometric Function2/1 -> Product8/1, Product8/3, Product8/2
  Divide2/1 -> Trigonometric Function1/1
  Divide1/1 -> Trigonometric Function/1
  Product7/1 -> Divide1/2
  Product6/1 -> Divide1/1
  Subtract2/1 -> Divide/1
  Product5/1 -> Divide/2, Subtract2/2
  Product4/1 -> Subtract2/1
  Gain/1 -> Subtract1/1
  Product3/1 -> Subtract1/2
  Sqrt/1 -> [P]
  Add/1 -> Sqrt/1
  Product2/1 -> Add/2
  Product1/1 -> Add/1
  Product/1 -> [b]
  Subtract/1 -> Product/2
  Constant/1 -> Subtract/1
  Trigonometric Function1/1 -> lat/1  "lat"
  [a] -> Product11/2
  Subtract1/1 -> Product11/1
  [P] -> Subtract3/1
  [b] -> Product10/2
  [z] -> Add1/1
  [b] -> Product7/2
  [P] -> Product7/1
  Trigonometric Function/1 -> Trigonometric Function2/1, Trigonometric Function3/1
  [a] -> Product6/2
  [z] -> Product6/1
  [f] -> Gain/1, Product3/1, Product3/2
  [b] -> Product5/1, Product5/2
  [a] -> Product4/1, Product4/2
  Demux1/2 -> Product2/1, Product2/2
  Demux1/1 -> Product1/1, Product1/2
  [f] -> Subtract/2
  [a] -> Product/1
  Demux1/3 -> [z]
  pBEE/1 -> Demux1/1
  c_rsma/1 -> [a]
  c_flat/1 -> [f]

== system test_GRM_Airframe/GRM_Airframe/aerodynamics/aerodynamic_via_lookup/calc_aero_for_mom/launch_rail1/initial_altitude/trafo_E_to_geodetic/Geodetic_altitude ==
  pBEE : Inport
  c_rsma : Inport  Port=2
  c_flat : Inport  Port=3
  lat : Inport  Port=4
  Add : Sum
  Constant : Constant
  Gain : Gain  Gain=2
  Product : Product  Inputs=*/  SaturateOnIntegerOverflow=on  RndMeth=Zero  InputSameDT=on  OutDataTypeStr=Inherit: Same as first input
  Product1 : Product
  Product2 : Product
  Product3 : Product
  Product4 : Product  Inputs=*/  SaturateOnIntegerOverflow=on  RndMeth=Zero  InputSameDT=on  OutDataTypeStr=Inherit: Same as first input
  Product5 : Product  Inputs=3
  Selector : Selector  IndexMode=Zero-based  InputPortWidth=3  IndexOptions=Index vector (dialog)  Indices=0  OutputSizes=1
  Selector1 : Selector  IndexMode=Zero-based  InputPortWidth=3  IndexOptions=Index vector (dialog)  Indices=1  OutputSizes=1
  Sqrt : Sqrt  SaturateOnIntegerOverflow=on
  Sqrt1 : Sqrt  SaturateOnIntegerOverflow=on
  Subtract : Sum  Inputs=+-
  Subtract1 : Sum  Inputs=+-
  Sum : Sum  Inputs=+-  SaturateOnIntegerOverflow=on  InputSameDT=on  OutDataTypeStr=Inherit: Same as first input
  Trigonometric Function : Trigonometry
  cos(latGD) : Trigonometry  Operator=cos
  alt : Outport  VectorParamsAs1DForOutWhenUnconnected=off
  wires:
  Product4/1 -> Sum/2
  Trigonometric Function/1 -> Product5/1, Product5/2
  Product5/1 -> Subtract1/2
  Constant/1 -> Subtract1/1
  Subtract1/1 -> Sqrt1/1
  Sqrt1/1 -> Product4/2
  c_flat/1 -> Gain/1, Product3/2, Product3/1
  Gain/1 -> Subtract/1
  Product3/1 -> Subtract/2
  pBEE/1 -> Selector/1, Selector1/1
  Add/1 -> Sqrt/1
  Product2/1 -> Add/2
  Product1/1 -> Add/1
  Selector1/1 -> Product2/1, Product2/2
  Selector/1 -> Product1/1, Product1/2
  Sum/1 -> alt/1  "alt"
  Product/1 -> Sum/1
  Subtract/1 -> Product5/3
  c_rsma/1 -> Product4/1
  cos(latGD)/1 -> Product/2
  Sqrt/1 -> Product/1
  lat/1 -> cos(latGD)/1, Trigonometric Function/1

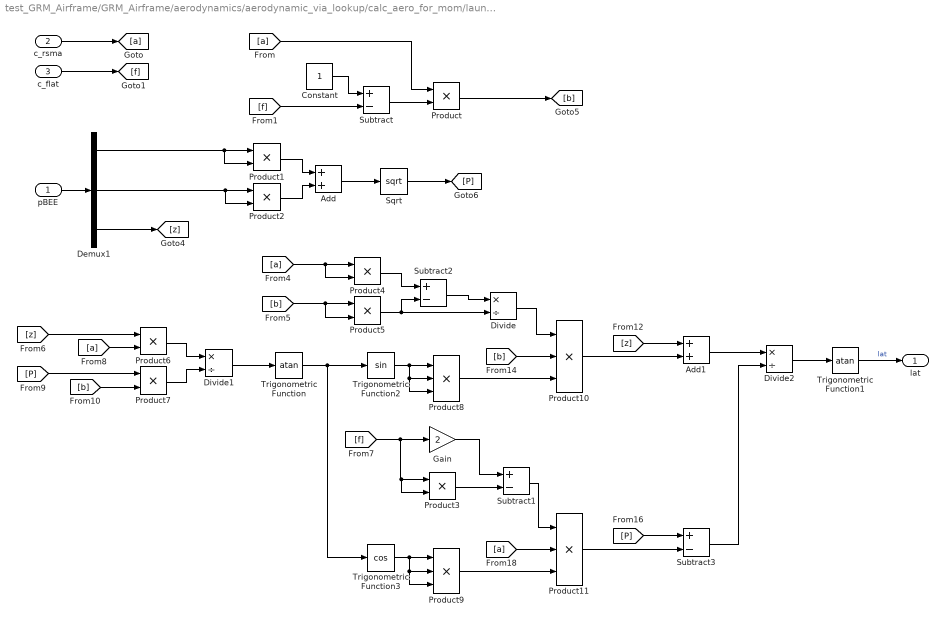
== system test_GRM_Airframe/GRM_Airframe/aerodynamics/aerodynamic_via_lookup/calc_aero_for_mom/launch_rail1/initial_altitude/trafo_E_to_geodetic/Geodetic_latitude ==
  pBEE : Inport
  c_rsma : Inport  Port=2
  c_flat : Inport  Port=3
  Add : Sum
  Add1 : Sum
  Constant : Constant
  Demux1 : Demux  Outputs=[1;1;1]
  Divide : Product  Inputs=*/
  Divide1 : Product  Inputs=*/
  Divide2 : Product  Inputs=*/
  Gain : Gain  Gain=2
  Product{,1..7} (8 alike) : Product
  Product{8..11} (4 alike) : Product  Inputs=3
  Sqrt : Sqrt  SaturateOnIntegerOverflow=on
  Subtract{,1..3} (4 alike) : Sum  Inputs=+-
  Trigonometric Function : Trigonometry  Operator=atan
  Trigonometric Function1 : Trigonometry  Operator=atan
  Trigonometric Function2 : Trigonometry
  Trigonometric Function3 : Trigonometry  Operator=cos
  lat : Outport  VectorParamsAs1DForOutWhenUnconnected=off
  wires:
  Divide/1 -> Product10/1
  Product9/1 -> Product11/3
  Product11/1 -> Subtract3/2
  Subtract3/1 -> Divide2/2
  Add1/1 -> Divide2/1
  Product10/1 -> Add1/2
  Product8/1 -> Product10/3
  Trigonometric Function3/1 -> Product9/1, Product9/3, Product9/2
  Trigonometric Function2/1 -> Product8/1, Product8/3, Product8/2
  Divide2/1 -> Trigonometric Function1/1
  Divide1/1 -> Trigonometric Function/1
  Product7/1 -> Divide1/2
  Product6/1 -> Divide1/1
  Subtract2/1 -> Divide/1
  Product5/1 -> Divide/2, Subtract2/2
  Product4/1 -> Subtract2/1
  Gain/1 -> Subtract1/1
  Product3/1 -> Subtract1/2
  Sqrt/1 -> [P]
  Add/1 -> Sqrt/1
  Product2/1 -> Add/2
  Product1/1 -> Add/1
  Product/1 -> [b]
  Subtract/1 -> Product/2
  Constant/1 -> Subtract/1
  Trigonometric Function1/1 -> lat/1  "lat"
  [a] -> Product11/2
  Subtract1/1 -> Product11/1
  [P] -> Subtract3/1
  [b] -> Product10/2
  [z] -> Add1/1
  [b] -> Product7/2
  [P] -> Product7/1
  Trigonometric Function/1 -> Trigonometric Function2/1, Trigonometric Function3/1
  [a] -> Product6/2
  [z] -> Product6/1
  [f] -> Gain/1, Product3/1, Product3/2
  [b] -> Product5/1, Product5/2
  [a] -> Product4/1, Product4/2
  Demux1/2 -> Product2/1, Product2/2
  Demux1/1 -> Product1/1, Product1/2
  [f] -> Subtract/2
  [a] -> Product/1
  Demux1/3 -> [z]
  pBEE/1 -> Demux1/1
  c_rsma/1 -> [a]
  c_flat/1 -> [f]

== matlab function test_GRM_Airframe/GRM_Airframe/aerodynamics/logic_base_drag/MATLAB Function ==
  data: u input; flag_base_drag output; t_prp2 input
function flag_base_drag = fcn(u, t_prp2)
%#codegen
if u >= 0 && u <= t_prp2 
    y = 0;
else
    y = 1;
    
end
flag_base_drag = y;

== matlab function test_GRM_Airframe/GRM_Airframe/fin_actuators/Rudder1/Limiting_Acceleration ==
  data: siB input; dd_siB_l output; d_siB input; dd_siB input; siB_min parameter; siB_max parameter; d_siB_min parameter; d_siB_max parameter; dd_siB_min parameter; dd_siB_max parameter
function dd_siB_l   = fcn(siB, d_siB, dd_siB, siB_min, siB_max, d_siB_min, d_siB_max, dd_siB_min, dd_siB_max)
%#codegen

%%   
dd_siB_l = dd_siB;

if dd_siB < dd_siB_min
    dd_siB_l = dd_siB_min;

elseif dd_siB_max < dd_siB
    dd_siB_l = dd_siB_max;
end;

if (siB <= siB_min && d_siB < 0) || (siB_max <= siB && 0 < d_siB)
    dd_siB_l = 0;
end;

if (d_siB <= d_siB_min && dd_siB < 0) || (d_siB_max <= d_siB && 0 < dd_siB)
    dd_siB_l = 0;
end

== matlab function test_GRM_Airframe/GRM_Airframe/environment/WGS84_Gravitation/WGS84_Gravity_Implementation ==
  data: pE input; lat_rad input; long_rad input; gamma_R output; c_rsma parameter; c_b_WGS parameter; c_grav parameter; c_rot parameter; flg_omega_enabled parameter
% Nach dem WGS84 Standard implementierte Gravitationsbeschleunigung 
%
% INPUTS:    
%   MANDATORY:
%       pE          ....... Positionsvektor im ECEF System
%       c_rsma      ....... Große Halbachse des WGS84 Ellipsoids
%       c_b_WGS     ....... Kleine Halbachse des WGS84 Ellipsoids
%       c_grav      ....... Gravitationskonstante der Erde nach WGS84
%       c_rot       ....... Rotationsgeschwindigkeit der Erde nach WGS84
%       flg_omega_enabled . Flag, die bestimmt ob die Rotation der Erde
%                           mitberechnet wird.
% 
% OUTPUTS:   
%       gamma_h     ....... Betrag des Gravitationsvektors
% 
% ABSTRACT: 
% Berechnet den absoluten Gravitationsbeschleunigungsbetrag nach Formel 4-4
% bis 4-13 des WGS84 Standards ( Technical Report
% "Department of Defense World Geodetic System 1984", NIMA TR8350.2,
% Third Edition, Amendment 1 vom 3 Januar 2000)
% 
%
% PROJECT:
%              *** GENERIC INTERCEPTOR SIMULATION ***
%
% REFERENCES:
% Technical Report
% "Department of Defense World Geodetic System 1984", NIMA TR8350.2,
% Third Edition, Amendment 1 vom 3 Januar 2000
%
% CHANGE LOG
% Date          Name                Description                     Version
% 2016.08.24    Philippe Petit      Inital Version                  V1.0
% 2016.11.16    Philippe Petit      Ausgabe der Gravitation als     V1.1
%                                   Vektor
% 2017.03.08    Christian Heise     Korrektur der Ausgabe, so dass  V1.2
%                                   wirklich ein Vektor im ECEF-
%                                   Frame zurückgegeben wird.

function gamma_R = wgs84_normalgravity(pE, lat_rad, long_rad, c_rsma, c_b_WGS, c_grav, c_rot, flg_omega_enabled)
%WGS84 Gravity Implementation
% a = 6378137.0;                  %[m], WGS84 Semi-major Axis 
% b = 6356752.3142;               %[m], WGS84 Semi-minor Axis
% omega = 7292115.8553e-11;       %[rad/s], WGS84 Angular Velocity of the Earth
% GM = 3986004.418e8;             %[m^3/s^2], Earths, Gravitational Constant
a       = c_rsma;
b       = c_b_WGS;
omega   = c_rot;
GM      = c_grav;
phi     = lat_rad;
lambda  = long_rad;

if norm(pE) < b
    error('Radius kleiner als die kleine halbachse...')
end

%Parse den Positionsvektor
x = pE(1);
y = pE(2);
z = pE(3);

%Formel 4-7 bis 4-13
E       = sqrt(a^2 - b^2);
u       = sqrt(1/2*(x^2+y^2+z^2-E^2)*(1+sqrt( 1 + (4*E^2*z^2)/(x^2+y^2+z^2-E^2)^2) ) );
beta    = atan2( z*sqrt(u^2+E^2) , u*sqrt(x^2+y^2) );
w       = sqrt((u^2 + E^2*sin(beta)^2)/(u^2 + E^2));
q       = 1/2*((1+3*u^2/E^2)*atan2(E,u)-3*u/E);
q_0     = 1/2*((1+3*b^2/E^2)*atan2(E,b)-3*b/E);
q_dash  = 3*(1+u^2/E^2)*(1-u/E*atan2(E,u))-1;

%Formel 4-5 und 4-6
gamma_u     = -1/w*( GM/(u^2+E^2) + omega^2*a^2*E/(u^2 + E^2)*q_dash/q_0*(1/2*sin(beta)^2 - 1/6) ) + flg_omega_enabled*1/w*omega^2*u*cos(beta)^2;
gamma_beta  = 1/w*omega^2*a^2/(u^2 + E^2)*q/q_0*sin(beta)*cos(beta) - flg_omega_enabled*1/w*omega^2*sqrt(u^2 + E^2) *sin(beta)*cos(beta);
gamma_lambda = 0;

%Formel 4-18 & 4-19
R1  = [u/(w*sqrt(u^2 + E^2))*cos(beta)*cos(lambda), -1/w*sin(beta)*cos(lambda), -sin(lambda);...                                      %Element(1,3)
       u/(w*sqrt(u^2 + E^2))*cos(beta)*sin(lambda), -1/w*sin(beta)*sin(lambda),  cos(lambda);...
       1/w*sin(beta)                              , u/(w*sqrt(u^2 + E^2))*cos(beta), 0];
% R2  = [cos(phi)*cos(lambda), cos(phi)*sin(lambda), sin(phi);...
%       -sin(phi)*cos(lambda), -sin(phi)*sin(lambda), cos(phi);...
%       -sin(lambda), cos(lambda), 0];
  
%Formel 4-16
gamma_E = [gamma_u; gamma_beta; gamma_lambda];
gamma_R = R1*gamma_E;

== matlab function test_GRM_Airframe/GRM_Airframe/fin_actuators/Rudder1/Limiting_Rate ==
  data: siB input; d_siB_l output; d_siB input; siB_min parameter; siB_max parameter; d_siB_min parameter; d_siB_max parameter
function d_siB_l  = fcn(siB, d_siB, siB_min, siB_max, d_siB_min, d_siB_max)
%#codegen

%%  
d_siB_l = d_siB;

if d_siB < d_siB_min
    d_siB_l = d_siB_min;
    
elseif d_siB_max < d_siB
    d_siB_l = d_siB_max;
    
end

 if (siB <= siB_min && d_siB < 0) || (siB_max <= siB && 0 < d_siB)
    d_siB_l = 0;
 end

== matlab function test_GRM_Airframe/GRM_Airframe/fin_actuators/Rudder2/Limiting_Acceleration ==
  data: siB input; dd_siB_l output; d_siB input; dd_siB input; siB_min parameter; siB_max parameter; d_siB_min parameter; d_siB_max parameter; dd_siB_min parameter; dd_siB_max parameter
function dd_siB_l   = fcn(siB, d_siB, dd_siB, siB_min, siB_max, d_siB_min, d_siB_max, dd_siB_min, dd_siB_max)
%#codegen

%%   
dd_siB_l = dd_siB;

if dd_siB < dd_siB_min
    dd_siB_l = dd_siB_min;

elseif dd_siB_max < dd_siB
    dd_siB_l = dd_siB_max;
end;

if (siB <= siB_min && d_siB < 0) || (siB_max <= siB && 0 < d_siB)
    dd_siB_l = 0;
end;

if (d_siB <= d_siB_min && dd_siB < 0) || (d_siB_max <= d_siB && 0 < dd_siB)
    dd_siB_l = 0;
end

== matlab function test_GRM_Airframe/GRM_Airframe/fin_actuators/Rudder/Limiting_Acceleration ==
  data: siB input; dd_siB_l output; d_siB input; dd_siB input; siB_min parameter; siB_max parameter; d_siB_min parameter; d_siB_max parameter; dd_siB_min parameter; dd_siB_max parameter
function dd_siB_l   = fcn(siB, d_siB, dd_siB, siB_min, siB_max, d_siB_min, d_siB_max, dd_siB_min, dd_siB_max)
%#codegen

%%   
dd_siB_l = dd_siB;

if dd_siB < dd_siB_min
    dd_siB_l = dd_siB_min;

elseif dd_siB_max < dd_siB
    dd_siB_l = dd_siB_max;
end;

if (siB <= siB_min && d_siB < 0) || (siB_max <= siB && 0 < d_siB)
    dd_siB_l = 0;
end;

if (d_siB <= d_siB_min && dd_siB < 0) || (d_siB_max <= d_siB && 0 < dd_siB)
    dd_siB_l = 0;
end

== matlab function test_GRM_Airframe/GRM_Airframe/fin_actuators/Rudder/Limiting_Rate ==
  data: siB input; d_siB_l output; d_siB input; siB_min parameter; siB_max parameter; d_siB_min parameter; d_siB_max parameter
function d_siB_l  = fcn(siB, d_siB, siB_min, siB_max, d_siB_min, d_siB_max)
%#codegen

%%  
d_siB_l = d_siB;

if d_siB < d_siB_min
    d_siB_l = d_siB_min;
    
elseif d_siB_max < d_siB
    d_siB_l = d_siB_max;
    
end

 if (siB <= siB_min && d_siB < 0) || (siB_max <= siB && 0 < d_siB)
    d_siB_l = 0;
 end

== matlab function test_GRM_Airframe/GRM_Airframe/fin_actuators/Rudder2/Limiting_Rate ==
  data: siB input; d_siB_l output; d_siB input; siB_min parameter; siB_max parameter; d_siB_min parameter; d_siB_max parameter
function d_siB_l  = fcn(siB, d_siB, siB_min, siB_max, d_siB_min, d_siB_max)
%#codegen

%%  
d_siB_l = d_siB;

if d_siB < d_siB_min
    d_siB_l = d_siB_min;
    
elseif d_siB_max < d_siB
    d_siB_l = d_siB_max;
    
end

 if (siB <= siB_min && d_siB < 0) || (siB_max <= siB && 0 < d_siB)
    d_siB_l = 0;
 end

== matlab function test_GRM_Airframe/GRM_Airframe/fin_actuators/Rudder3/Limiting_Acceleration ==
  data: siB input; dd_siB_l output; d_siB input; dd_siB input; siB_min parameter; siB_max parameter; d_siB_min parameter; d_siB_max parameter; dd_siB_min parameter; dd_siB_max parameter
function dd_siB_l   = fcn(siB, d_siB, dd_siB, siB_min, siB_max, d_siB_min, d_siB_max, dd_siB_min, dd_siB_max)
%#codegen

%%   
dd_siB_l = dd_siB;

if dd_siB < dd_siB_min
    dd_siB_l = dd_siB_min;

elseif dd_siB_max < dd_siB
    dd_siB_l = dd_siB_max;
end;

if (siB <= siB_min && d_siB < 0) || (siB_max <= siB && 0 < d_siB)
    dd_siB_l = 0;
end;

if (d_siB <= d_siB_min && dd_siB < 0) || (d_siB_max <= d_siB && 0 < dd_siB)
    dd_siB_l = 0;
end

== matlab function test_GRM_Airframe/GRM_Airframe/fin_actuators/Rudder3/Limiting_Rate ==
  data: siB input; d_siB_l output; d_siB input; siB_min parameter; siB_max parameter; d_siB_min parameter; d_siB_max parameter
function d_siB_l  = fcn(siB, d_siB, siB_min, siB_max, d_siB_min, d_siB_max)
%#codegen

%%  
d_siB_l = d_siB;

if d_siB < d_siB_min
    d_siB_l = d_siB_min;
    
elseif d_siB_max < d_siB
    d_siB_l = d_siB_max;
    
end

 if (siB <= siB_min && d_siB < 0) || (siB_max <= siB && 0 < d_siB)
    d_siB_l = 0;
 end
